simulink model "sim_bandpass_singleBand"  (R2020a)
settings: Solver=FixedStepDiscrete  StartTime=0.0  StopTime=(size(sm_EEG_data,1)-1)/sm.p.EEG.sr  RelTol=1e-3  EnableMultiTasking=on
undefined symbols (not defined in the file or in its folder): fdesignblkfcn, gcbh, sm
libraries: dspsrcs4 x1
settings Model: Creator=ronens  LastModifiedBy=Rober
settings DataIOCC: LimitDataPoints=on  SaveFormat=Array  SignalLoggingSaveFormat=ModelDataLogs  ReturnWorkspaceOutputs=off
settings OptimizationCC: ExpressionDepthLimit=2147483647  LifeSpan=inf
settings DebuggingCC: UnderspecifiedInitializationDetection=Classic  MergeDetectMultiDrivingBlocksExec=none  SolverPrmCheckMsg=warning  ParameterPrecisionLossMsg=none  FcnCallInpInsideContextMsg=warning  StateNameClashWarn=warning  SFUnexpectedBacktrackingDiag=warning  SFNoUnconditionalDefaultTransitionDiag=warning  SFExecutionAtInitializationDiag=none  ArithmeticOperatorsInVariantConditions=warning
settings HardwareCC: ProdBitPerPointer=32  ProdBitPerSizeT=32  ProdBitPerPtrDiffT=32  ProdLargestAtomicFloat=None  ProdIntDivRoundTo=Undefined  ProdEndianess=Unspecified  ProdWordSize=32  ProdHWDeviceType=32-bit Generic
settings ModelReferenceCC: PropagateSignalLabelsOutOfModel=off
settings SFSimCC: SimUseLocalCustomCode=off  CustomCodeUndefinedFunction=UseInterfaceOnly
settings RTWCC: RTWUseLocalCustomCode=off
settings CodeAppCC: StateflowObjectComments=on
settings GRTTargetCC: TargetLangStandard=C89/C90 (ANSI)
settings ConfigComp: CovMetricSettings=dw  CovSaveCumulativeToWorkspaceVar=on  CovSaveSingleToWorkspaceVar=on  CovExternalEMLEnable=off
settings ConfigurationSet: Description=SimMechanics 2G

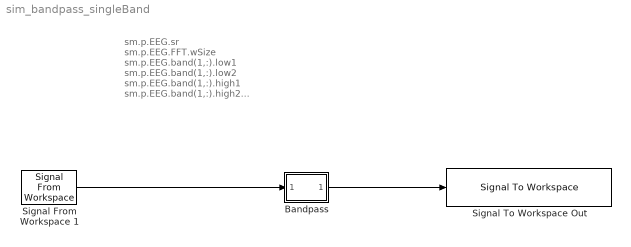
== system sim_bandpass_singleBand ==
  note: sm.p.EEG.sr
      | sm.p.EEG.FFT.wSize
      | sm.p.EEG.band(1,:).low1
      | sm.p.EEG.band(1,:).low2
      | sm.p.EEG.band(1,:).high1
      | sm.p.EEG.band(1,:).high2
      | sm.p.EEG.band_stop_dB
      | sm.p.EEG.band_pass_dB
  Bandpass : Subsystem
  Signal From Workspace 1 : dspsrcs4/Signal From Workspace  X=sm_EEG_data  Ts=1/sm.p.EEG.sr  nsamps=1  OutputAfterFinalValue=Setting to zero  ignoreOrWarnInputAndFrameLengths=off  OutputFrames=on
  Signal To Workspace Out : SignalToWorkspace  VariableName=Bandpass_singleBand
      settings: CopyFcn=dspblkcopystw(gcbh);
  wires:
  Signal From Workspace 1/1 -> Bandpass/1(In1)
  Bandpass/1(Out1) -> Signal To Workspace Out/1

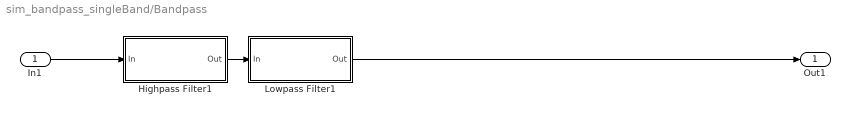
== system sim_bandpass_singleBand/Bandpass ==
  In1 : Inport
  Highpass Filter1 : Subsystem  DialogController=fdesignblkfcn  InitFcn=fdesignblkfcn(gcbh, {'InitFcn'});  mask(Highpass Filter){}
      mask help: Design a highpass filter
      settings: CopyFcn=fdesignblkfcn(gcbh, {'CopyFcn'});
      mask Help: helpview(mapfilelocation('dsp'), 'dsphighpassfilter');
      mask Display: disp('Highpass')
  Lowpass Filter1 : Subsystem  DialogController=fdesignblkfcn  InitFcn=fdesignblkfcn(gcbh, {'InitFcn'});  mask(Lowpass Filter){}
      mask help: Design a lowpass filter
      settings: CopyFcn=fdesignblkfcn(gcbh, {'CopyFcn'});
      mask Help: helpview(mapfilelocation('dsp'), 'dsplowpassfilter');
      mask Display: disp('Lowpass')
  Out1 : Outport
  wires:
  In1/1 -> Highpass Filter1/1(In)
  Highpass Filter1/1(Out) -> Lowpass Filter1/1(In)
  Lowpass Filter1/1(Out) -> Out1/1

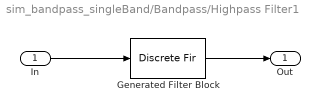
== system sim_bandpass_singleBand/Bandpass/Highpass Filter1 ==
  In : Inport
  Generated Filter Block : DiscreteFir  Tag=BlockMethodSubSystem  Coefficients=[-0.00909138480974088121 0.0151910446097941066 0.00203287238871485655 -0.00378447045136760156 -0.00516212061084350606 -0.00394998824205581352 -0.00138475812735488427 0.00149221871062396377 0.00373920873979393569 0.00453767723231078036 0.0035033798033534307 0.000891058924022470971 -0.00240102635565997728 -0.00504825972126061312 -0.0058140559906373554 -0.00411215037222385869 -0.000342694321446404809 0.00411796966931580067 0.00738259459742753119 0.00781480904310332368 0.00481740783652252671 -0.00076736960812694632 -0.00683697228361345756 -0.0107654861902180595 -0.0104852866066524903 -0.00548353883209012904 0.00275843011748880609 0.011098143756347113 0.015844631795687094 0.0142844273503884046 0.00603685108990855736 -0.00642265895848751368 -0.0183705391674457083 -0.0244077606940095206 -0.0206037711332415809 -0.00646406920455855349 0.0141939545539890074 0.0339016637956632838 0.0436387040915278551 0.0357238367352588349 0.00672576511710388028 -0.0407004687071831003 -0.0980849407850058058 -0.153002565135390622 -0.192453144900027767 0.793158879366609337 -0.192453144900027767 -0.153002565135390622 -0.0980849407850058058 -0.0407004687071831003 0.00672576511710388028 0.0357238367352588349 0.0436387040915278551 0.0339016637956632838 0.0141939545539890074 -0.00646406920455855349 -0.0206037711332415809 -0.0244077606940095206 -0.0183705391674457083 -0.00642265895848751368 0.00603685108990855736 0.0142844273503884046 0.015844631795687094 0.011098143756347113 0.00275843011748880609 -0.00548353883209012904 -0.0104852866066524903 -0.0107654861902180595 -0.00683697228361345756 -0.00076736960812694632 0.00481740783652252671 0.00781480904310332368 0.00738259459742753119 0.00411796966931580067 -0.000342694321446404809 -0.00411215037222385869 -0.0058140559906373554 -0.00504825972126061312 -0.00240102635565997728 0.000891058924022470971 0.0035033798033534307 0.00453767723231078036 0.00373920873979393569 0.00149221871062396377 -0.00138475812735488427 -0.00394998824205581352 -0.00516212061084350606 -0.00378447045136760156 0.00203287238871485655 0.0151910446097941066 -0.00909138480974088121]  InputProcessing=Columns as channels (frame based)
  Out : Outport
  wires:
  Generated Filter Block/1 -> Out/1
  In/1 -> Generated Filter Block/1

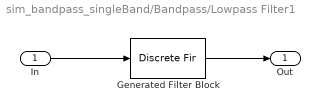
== system sim_bandpass_singleBand/Bandpass/Lowpass Filter1 ==
  In : Inport
  Generated Filter Block : DiscreteFir  Tag=BlockMethodSubSystem  Coefficients=[0.000856440286467256146 -0.000224538909107539287 -0.00355374838699149161 -0.00850375078310230612 -0.0116575787622561315 -0.00945245496276940142 -0.00198623838759905483 0.00566292802366960037 0.0071060127473432334 0.000849790511033779537 -0.00712986290885135859 -0.008284206561930808 -0.00022369873952942515 0.0095712967638715684 0.0102833065448347111 -0.000670874450634086593 -0.013070216771608658 -0.0129489859101078464 0.00220475618195314742 0.0181353437580406666 0.016528784950566193 -0.00484871103652279728 -0.0258418171641096039 -0.0216755167547303118 0.00970543171364747666 0.0391099748818777709 0.0304843043055294527 -0.0201080643459090568 -0.0686819810823017518 -0.0524462558227782039 0.055242910080728902 0.211511848633576693 0.326100954586855174 0.326100954586855174 0.211511848633576693 0.055242910080728902 -0.0524462558227782039 -0.0686819810823017518 -0.0201080643459090568 0.0304843043055294527 0.0391099748818777709 0.00970543171364747666 -0.0216755167547303118 -0.0258418171641096039 -0.00484871103652279728 0.016528784950566193 0.0181353437580406666 0.00220475618195314742 -0.0129489859101078464 -0.013070216771608658 -0.000670874450634086593 0.0102833065448347111 0.0095712967638715684 -0.00022369873952942515 -0.008284206561930808 -0.00712986290885135859 0.000849790511033779537 0.0071060127473432334 0.00566292802366960037 -0.00198623838759905483 -0.00945245496276940142 -0.0116575787622561315 -0.00850375078310230612 -0.00355374838699149161 -0.000224538909107539287 0.000856440286467256146]  InputProcessing=Columns as channels (frame based)
  Out : Outport
  wires:
  In/1 -> Generated Filter Block/1
  Generated Filter Block/1 -> Out/1
